simulink model "srm_test_2012"  (R2012b)
settings: Solver=ode45  SolverMode=SingleTasking  StartTime=0.0  StopTime=1.0  RelTol=1e-3
undefined symbols (not defined in the file): DiscIntNeverNeededParam
libraries: powerlib x15
settings Model: CovMetricSettings=dwe  CovHtmlReporting=off  covSaveCumulativeToWorkspaceVar=off  CovSaveSingleToWorkspaceVar=off  CovExternalEMLEnable=on  Creator=DELL  LastModifiedBy=DELL
settings DataIOCC: LimitDataPoints=off  SaveFormat=StructureWithTime  ReturnWorkspaceOutputs=on
settings OptimizationCC: ExpressionDepthLimit=128
settings DebuggingCC: UnderspecifiedInitializationDetection=Simplified  MergeDetectMultiDrivingBlocksExec=error  SolverPrmCheckMsg=none  FrameProcessingCompatibilityMsg=error  StateNameClashWarn=none  SFUnexpectedBacktrackingDiag=error  SFNoUnconditionalDefaultTransitionDiag=error
settings HardwareCC: ProdBitPerPointer=64  ProdLargestAtomicFloat=Float  ProdIntDivRoundTo=Zero  ProdEndianess=LittleEndian  ProdHWDeviceType=Specified
settings ModelReferenceCC: PropagateSignalLabelsOutOfModel=on
settings SFSimCC: SimUseLocalCustomCode=on
settings RTWCC: RTWUseLocalCustomCode=on
settings CodeAppCC: CustomSymbolStrType=$N$R$M_T
settings GRTTargetCC: CodeReplacementLibrary=C99 (ISO)  GeneratePreprocessorConditionals=Use local settings

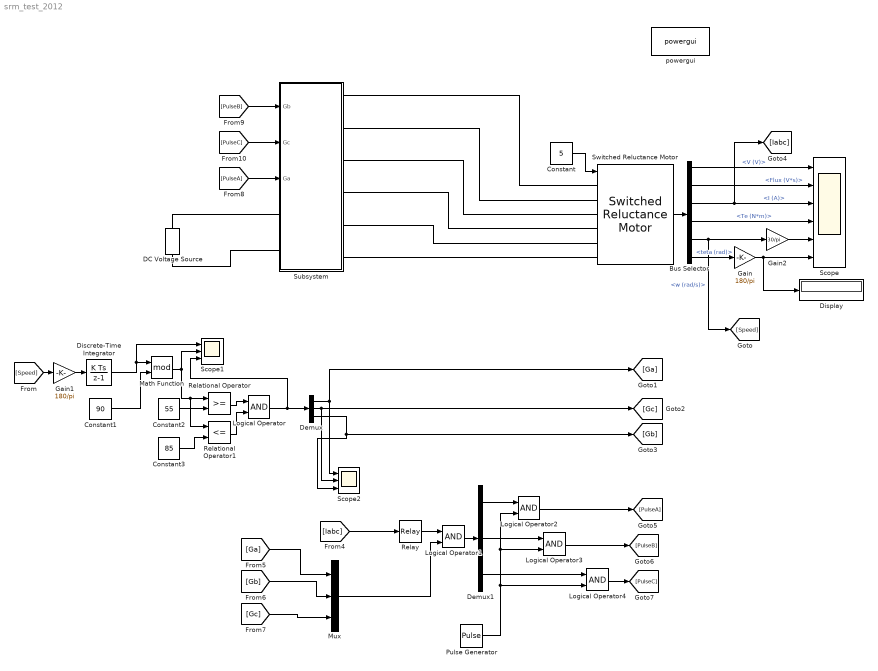
== system srm_test_2012 ==
  Bus Selector : BusSelector  OutputSignals=V (V),Flux (V*s),I (A),Te (N*m),w (rad/s),teta (rad)
  Constant : Constant  Value=5
  Constant1 : Constant  Value=90
  Constant2 : Constant  Value=55
  Constant3 : Constant  Value=85
  DC Voltage Source : powerlib/Electrical Sources/DC Voltage Source  Amplitude=72  Measurements=None
  Demux : Demux  Outputs=3
  Demux1 : Demux  Outputs=3
  Discrete-Time Integrator : DiscreteIntegrator  InitialCondition=[0 30 60]  InitialConditionMode=State only (most efficient)  SampleTime=10e-6  ICPrevOutput=DiscIntNeverNeededParam  ICPrevScaledInput=DiscIntNeverNeededParam
  Display : Display
  Gain : Gain  Gain=180/pi
  Gain1 : Gain  Gain=180/pi
  Gain2 : Gain  Gain=30/pi
  Logical Operator{,1..4} (5 alike) : Logic  AllPortsSameDT=off  OutDataTypeStr=boolean
  Math Function : Math  Operator=mod  SaturateOnIntegerOverflow=on
  Mux : Mux  Inputs=3
  Pulse Generator : DiscretePulseGenerator  PulseType=Time based  Period=1/5000  PulseWidth=90
  Relational Operator : RelationalOperator  OutDataTypeStr=boolean
  Relational Operator1 : RelationalOperator  Operator=<=  OutDataTypeStr=boolean
  Relay : Relay  OnSwitchValue=110  OffSwitchValue=80  OnOutputValue=0  OffOutputValue=1
  Scope : Scope  NumInputPorts=6
      settings: TimeRange=auto  MaxDataPoints=5000  SaveToWorkspace=off  SaveName=ScopeData  YMin=-219.56061~-0.05314~-15.19769~-10.34235~-147.73313~-546.25144  YMax=1218.92371~0.46646~126.29796~93.08117~1299.39502~4916.0217  SampleTime=-1
  Scope1 : Scope  NumInputPorts=3
      settings: TimeRange=auto  MaxDataPoints=5000  SaveToWorkspace=off  YMin=-309.77108~-11.24995~-0.125  YMax=2787.93973~101.24953~1.125  SampleTime=-1
  Scope2 : Scope  NumInputPorts=3
      settings: TimeRange=auto  MaxDataPoints=5000  SaveToWorkspace=off  SaveName=ScopeData2  YMin=-1.00000~-1.00000~0.9  YMax=1.00000~1.00000~1.1  SampleTime=-1
  Subsystem : Subsystem
  Switched Reluctance Motor : powerlib/Machines/Switched Reluctance Motor  MachineType=6/4  StatorResistance=0.01  Inertia=0.0082  Friction=0.01  InitialSpeed=[0 0]  TsPowergui=0  TsBlock=-1  MachineModel=Generic model  Lq=0.67e-3  Ld=23.6e-3  Lsat=0.15e-3  MaximumCurrent=450  MaximumFluxLinkage=0.486  Source=MAT-file  MagnetisationCharacteristic='srm64_60kw.mat'  RotorAngleVector=[0 10 20 30 40 45]  StatorCurrentVector=[0:25:450]  PlotCurves=off
  powergui : powerlib/powergui  Priority=1  SimulationMode=Discrete  SampleTime=10e-6  frequency=60  Iterations=50  frequencyindice=0  Pbase=100e6  ErrMax=1e-4  UnitsV=kV  UnitsW=MW  buscounter=0  FunctionMessages=off  echomessages=off  EnableUseOfTLC=off  CurrentSourceSwitches=off  DisableSnubberDevices=off  DisableRonSwitches=off  DisableVfSwitches=off  DisplayEquations=off  AutomaticDiscreteSolvers=off  SolverType=Tustin/Backward Euler (TBE)  Interpol=off  ExternalGateDelay=off  methode=off  Ts=100  x0status=blocks  SPID=on  SwTol=0  HookPort=off  NonlinearTolerance=1e-4  nMaxIteration=100  ContinueOnMaxIteration=off  RestoreLinks=warning  ResistiveCurrentMeasurement=off  Frange=[0:2:500]  Ylog=off  Xlog=on  ShowGrid=off  save=off  variable=ZData  structure=0  ZoomFFT=off  StartTime=0.0  cycles=1  DisplayStyle=1  fundamental=60  FreqAxis=off  MaxFrequency=1000  frequencyindicesteady=1  RmsSteady=1  display=off
  wires:
  Switched Reluctance Motor/1 -> Bus Selector/1
  Bus Selector/1 -> Scope/1  "<V (V)>"
  Bus Selector/2 -> Scope/2  "<Flux (V*s)>"
  Bus Selector/3 -> [Iabc], Scope/3  "<I (A)>"
  Bus Selector/4 -> Scope/4  "<Te (N*m)>"
  Bus Selector/5 -> [Speed], Gain2/1  "<w (rad/s)>"
  Bus Selector/6 -> Gain/1  "<teta (rad)>"
  Gain/1 -> Scope/6, Display/1
  [Speed] -> Gain1/1
  Gain1/1 -> Discrete-Time Integrator/1
  Discrete-Time Integrator/1 -> Math Function/1, Scope1/1
  Constant/1 -> Switched Reluctance Motor/1
  Constant1/1 -> Math Function/2
  Math Function/1 -> Relational Operator1/1, Relational Operator/1, Scope1/2
  Constant2/1 -> Relational Operator/2
  Constant3/1 -> Relational Operator1/2
  Relational Operator/1 -> Logical Operator/1
  Relational Operator1/1 -> Logical Operator/2
  Logical Operator/1 -> Demux/1, Scope1/3
  Demux/1 -> Scope2/1, [Ga]
  Demux/2 -> [Gc], Scope2/2
  Demux/3 -> Scope2/3, [Gb]
  [PulseA] -> Subsystem/3(Ga)
  [PulseC] -> Subsystem/2(Gc)
  [PulseB] -> Subsystem/1(Gb)
  Gain2/1 -> Scope/5
  [Iabc] -> Relay/1
  Relay/1 -> Logical Operator1/1
  [Ga] -> Mux/1
  [Gb] -> Mux/2
  [Gc] -> Mux/3
  Mux/1 -> Logical Operator1/2
  Logical Operator1/1 -> Demux1/1
  Demux1/1 -> Logical Operator2/1
  Logical Operator2/1 -> [PulseA]
  Demux1/2 -> Logical Operator3/1
  Demux1/3 -> Logical Operator4/1
  Pulse Generator/1 -> Logical Operator4/2, Logical Operator3/2, Logical Operator2/2
  Logical Operator4/1 -> [PulseC]
  Logical Operator3/1 -> [PulseB]
  connections:
  Subsystem/RConn1 -- Switched Reluctance Motor/LConn1
  Switched Reluctance Motor/LConn2 -- Subsystem/RConn2
  Subsystem/RConn3 -- Switched Reluctance Motor/LConn3
  DC Voltage Source/RConn1 -- Subsystem/LConn1
  Subsystem/RConn4 -- Switched Reluctance Motor/LConn4
  Subsystem/LConn2 -- DC Voltage Source/LConn1
  Subsystem/RConn5 -- Switched Reluctance Motor/LConn5
  Subsystem/RConn6 -- Switched Reluctance Motor/LConn6

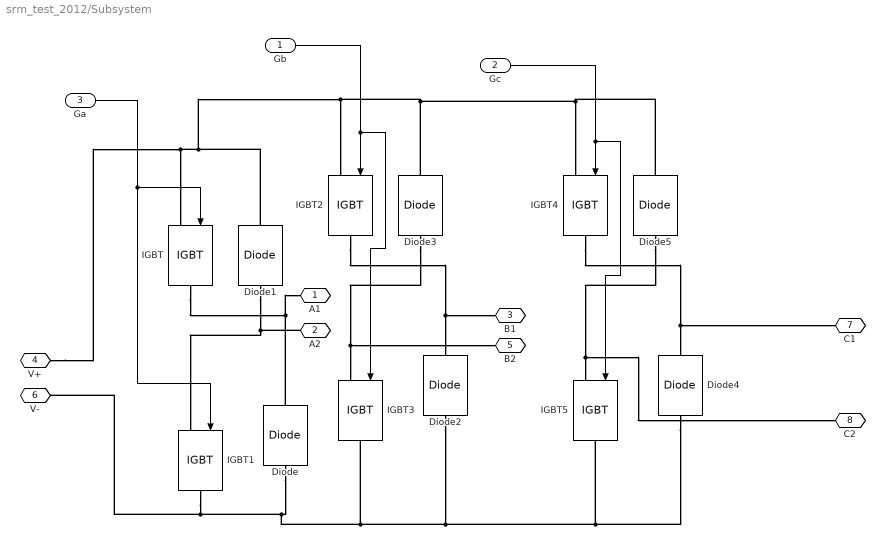
== system srm_test_2012/Subsystem ==
  Gb : Inport
  Gc : Inport  Port=2
  Ga : Inport  Port=3
  Diode{,1..5} (6 alike) : powerlib/Power Electronics/Diode  Ron=0.001  Lon=0  Vf=0.8  IC=0  UseSnubber=0  Rs=500  Cs=250e-9  Measurements=off
  IGBT{,1..5} (6 alike) : powerlib/Power Electronics/IGBT  Ron=0.001  Lon=0  Vf=1  Tf=1e-6  Tt=2e-6  IC=0  Rs=1e5  Cs=inf  Measurements=off
  A1 : PMIOPort  Side=Right
  A2 : PMIOPort  Port=2  Side=Right
  B1 : PMIOPort  Port=3  Side=Right
  V+ : PMIOPort  Port=4  Side=Left
  B2 : PMIOPort  Port=5  Side=Right
  V- : PMIOPort  Port=6  Side=Left
  C1 : PMIOPort  Port=7  Side=Right
  C2 : PMIOPort  Port=8  Side=Right
  wires:
  Gb/1 -> IGBT3/1, IGBT2/1
  Gc/1 -> IGBT5/1, IGBT4/1
  Ga/1 -> IGBT1/1, IGBT/1
  connections:
  Diode4/LConn1 -- Diode2/LConn1 -- V-/RConn1 -- IGBT1/RConn1 -- Diode/LConn1 -- IGBT3/RConn1 -- IGBT5/RConn1
  IGBT4/RConn1 -- C1/RConn1 -- Diode4/RConn1
  Diode5/RConn1 -- V+/RConn1 -- IGBT/LConn1 -- Diode1/RConn1 -- IGBT2/LConn1 -- Diode3/RConn1 -- IGBT4/LConn1
  Diode3/LConn1 -- IGBT3/LConn1 -- B2/RConn1
  Diode5/LConn1 -- C2/RConn1 -- IGBT5/LConn1
  IGBT2/RConn1 -- Diode2/RConn1 -- B1/RConn1
  IGBT/RConn1 -- Diode/RConn1 -- A1/RConn1
  Diode1/LConn1 -- IGBT1/LConn1 -- A2/RConn1
